simulink model "AC_FuzzyControl"  (R2020a)
settings: Solver=VariableStepAuto  StartTime=0.0  StopTime=1400  MaxStep=0.01  RelTol=1e-3  EnableMultiTasking=on
InitFcn:
  | R=4
  | C=3.6
  | Rm=1
  | Cm=4.3
  | eta=3
  | Tmin=19.5
  | Tmax=20.5
  | P=0.6
  | deltaT=2
libraries: simulink x2, fuzblock x1, dspstat3 x1
settings Model: Creator=daniel  LastModifiedBy=User
settings SolverCC: ZeroCrossControl=DisableAll
settings DataIOCC: LimitDataPoints=on  ReturnWorkspaceOutputs=off
settings OptimizationCC: LifeSpan=inf
settings DebuggingCC: AllowSymbolicDim=off  SFUnexpectedBacktrackingDiag=warning  SFNoUnconditionalDefaultTransitionDiag=warning  SFExecutionAtInitializationDiag=none  ArithmeticOperatorsInVariantConditions=warning
settings ModelReferenceCC: PropagateSignalLabelsOutOfModel=off
settings SFSimCC: SimUseLocalCustomCode=off  CustomCodeUndefinedFunction=UseInterfaceOnly
settings RTWCC: RTWUseLocalCustomCode=off
settings CodeAppCC: StateflowObjectComments=on
settings GRTTargetCC: TargetLangStandard=C89/C90 (ANSI)
settings ConfigComp: CovMetricSettings=dw  CovHtmlReporting=on  CovSaveCumulativeToWorkspaceVar=on  CovSaveSingleToWorkspaceVar=on  CovExternalEMLEnable=off

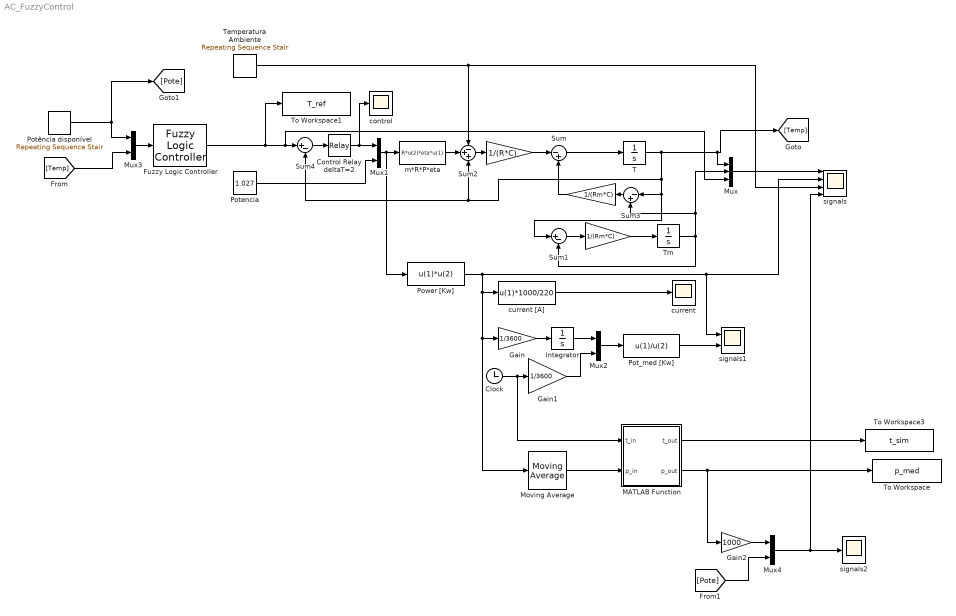
== system AC_FuzzyControl ==
  " " : Gain  Gain=1/(Rm*C)
  "  " : Gain  Gain=1/(Rm*C)
  "   " : Gain  Gain=1/(R*C)
  Clock : Clock
  Control Relay deltaT=2 : Relay  OnSwitchValue=0.5  OffSwitchValue=-0.5  OnOutputValue=0  OffOutputValue=1
  Fuzzy Logic Controller : fuzblock/Fuzzy Logic  Controller  FIS=AC_Fuzzy_neww  OutputSampleNumber=101  DataType=double  FuzzifiedInputs=off  RuleFiringStrengths=off  RuleOutputs=off  AggregatedOutputs=off  SimulateUsing=Interpreted execution  OutOfRangeInputValueMessage=warning  NoRuleFiredMessage=warning  EmptyOutputFuzzySetMessage=warning
  Gain : Gain  Gain=1/3600
  Gain1 : Gain  Gain=1/3600
  Gain2 : Gain  Gain=1000
  Integrator : Integrator
  MATLAB Function : MATLAB Function  TreatAsAtomicUnit=on
  Moving Average : dspstat3/Moving Average  Method=Sliding window  ForgettingFactorPort=off  SpecifyWindowLength=on  WindowLength=6000  ForgettingFactor=0.9  SimulateUsing=Code generation
  Mux : Mux  Inputs=3
  Mux{1..4} (4 alike) : Mux  Inputs=2
  Pot_med [Kw] : Fcn  Expr=u(1)/u(2)
  Potencia : Constant  Value=1.027
  Potência disponível : simulink/Sources/Repeating Sequence Stair  OutValues=[600 400 200]  tsamp=500  OutMin=[]  OutMax=[]  OutDataTypeStr=double  OutputDataTypeScalingMode=double  OutDataType=fixdt(0,8)  ConRadixGroup=Best Precision: Vector-wise  OutScaling=2^-12
  Power [Kw] : Fcn  Expr=u(1)*u(2)
  Sum : Sum  Inputs=|-+
  Sum1 : Sum  Inputs=|+-
  Sum2 : Sum  Inputs=-++
  Sum3 : Sum  Inputs=|-+
  Sum4 : Sum  Inputs=|+-
  T : Integrator  InitialCondition=30
  Temperatura Ambiente : simulink/Sources/Repeating Sequence Stair  OutValues=[32 30 25 20 15 10 5]  tsamp=200  OutMin=[]  OutMax=[]  OutDataTypeStr=double  OutputDataTypeScalingMode=double  OutDataType=fixdt(0,8)  ConRadixGroup=Best Precision: Vector-wise  OutScaling=2^-12
  Tm : Integrator  InitialCondition=30
  To Workspace : ToWorkspace  VariableName=p_med  SaveFormat=Timeseries  SampleTime=-1
  To Workspace1 : ToWorkspace  VariableName=T_ref  SaveFormat=Timeseries  SampleTime=-1
  To Workspace3 : ToWorkspace  VariableName=t_sim  SaveFormat=Timeseries  SampleTime=-1
  control : Scope
  "current " : Scope
  current [A] : Fcn  Expr=u(1)*1000/220
  m*R*P*eta : Fcn  Expr=R*u(2)*eta*u(1)
  signals : Scope  NumInputPorts=4
  signals1 : Scope  NumInputPorts=2
  signals2 : Scope
  wires:
  T/1 -> Sum1/1, Sum3/1, Sum4/2, Sum2/3, [Temp], Mux/1
  Sum/1 -> T/1
  "  "/1 -> Sum/2
  Sum1/1 -> " "/1
  " "/1 -> Tm/1
  Tm/1 -> Mux/2, Sum3/2, Sum1/2
  "   "/1 -> Sum/1
  Sum2/1 -> "   "/1
  Sum3/1 -> "  "/1
  m*R*P*eta/1 -> Sum2/2
  Mux/1 -> signals/1
  Sum4/1 -> Control Relay deltaT=2/1
  Fuzzy Logic Controller/1 -> To Workspace1/1, Mux/3, Sum4/1
  Temperatura Ambiente/1 -> signals/3, Sum2/1
  Potencia/1 -> Mux1/2
  Mux1/1 -> m*R*P*eta/1, Power [Kw]/1
  Control Relay deltaT=2/1 -> control/1, Mux1/1
  current [A]/1 -> "current "/1
  Power [Kw]/1 -> Moving Average/1, Gain/1, current [A]/1, signals1/1, signals/2
  Gain/1 -> Integrator/1
  Mux2/1 -> Pot_med [Kw]/1
  Clock/1 -> MATLAB Function/1(t_in), Gain1/1
  Gain1/1 -> Mux2/2
  Integrator/1 -> Mux2/1
  Pot_med [Kw]/1 -> signals1/2
  Moving Average/1 -> MATLAB Function/2(p_in)
  MATLAB Function/2(p_out) -> Gain2/1, To Workspace/1
  MATLAB Function/1(t_out) -> To Workspace3/1
  Potência disponível/1 -> Mux3/1, [Pote]
  [Temp] -> Mux3/2
  Mux3/1 -> Fuzzy Logic Controller/1
  [Pote] -> Mux4/2
  Gain2/1 -> Mux4/1
  Mux4/1 -> signals/4, signals2/1

== matlab function AC_FuzzyControl/MATLAB Function ==
  data: t_in input; t_out output; p_in input; p_out output
function [t_out,p_out] = fcn(t_in,p_in)

t_out=t_in;
p_out=p_in;
